simulink model "sl_subsys_trig1"  (Simulink 6.0)
settings: Solver=FixedStepDiscrete  SolverMode=SingleTasking  StartTime=0.0  StopTime=10.0  RelTol=1e-3
settings Model: CovMetricSettings=d  Creator=The MathWorks Inc.  LastModifiedBy=batserve  ExtModeAutoUpdateStatusClock=off
settings OptimizationCC: BlockReduction=off  BooleanDataType=off
settings DebuggingCC: CheckExecutionContextPreStartOutputMsg=on  CheckExecutionContextRuntimeOutputMsg=on  SolverPrmCheckMsg=none
settings HardwareCC: TargetUnknown=on

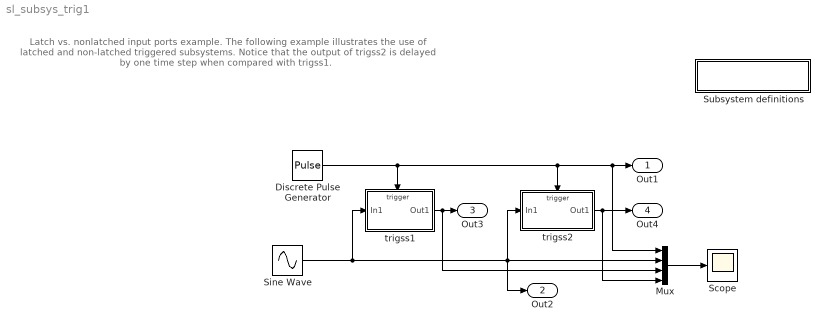
== system sl_subsys_trig1 ==
  note: Latch vs. nonlatched input ports example.
      |
      | The following example illustrates the use of latched
      | and non-latched triggered subsystems. Notice that
      | the output of trigss2 is delayed by one time step
      | when compared with trigss1.
  " Subsystem definitions" : Subsystem  PropExecContextAcrossSSBoundary=on
      settings: OpenFcn=helpview([matlabroot,'/toolbox/simulink/simdemos/sl_subsys_definitions.html']);
      mask Display: disp('Subsystem\ndefinitions')
  Discrete Pulse Generator : DiscretePulseGenerator
  Mux : Mux
  Scope : Scope
  Sine Wave : Sin  SineType=Sample based  Amplitude=2  Samples=20  SampleTime=.25
  trigss1 : Subsystem  TreatAsAtomicUnit=on  PropExecContextAcrossSSBoundary=on
  trigss2 : Subsystem  TreatAsAtomicUnit=on  PropExecContextAcrossSSBoundary=on
  Out1 : Outport
  Out2 : Outport  Port=2
  Out3 : Outport  Port=3
  Out4 : Outport  Port=4
  wires:
  trigss1/1(Out1) -> Out3/1, Mux/3
  trigss2/1(Out1) -> Out4/1, Mux/4
  Discrete Pulse Generator/1 -> trigss1/Trigger, trigss2/Trigger, Out1/1, Mux/1
  Sine Wave/1 -> trigss1/1(In1), trigss2/1(In1), Out2/1, Mux/2
  Mux/1 -> Scope/1

== system sl_subsys_trig1/ Subsystem definitions ==

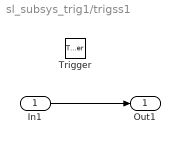
== system sl_subsys_trig1/trigss1 ==
  In1 : Inport  Port=1  LatchInput=off
  Trigger : TriggerPort
  Out1 : Outport
  wires:
  In1/1 -> Out1/1

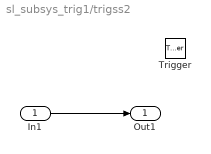
== system sl_subsys_trig1/trigss2 ==
  In1 : Inport  Port=1  LatchInput=on
  Trigger : TriggerPort
  Out1 : Outport
  wires:
  In1/1 -> Out1/1
